simulink model "demoOtterUSVPathFollowingCourseControl"  (R2021a)
settings: Solver=ode4  StartTime=0.0  StopTime=300  FixedStep=0.05  RelTol=1e-3
libraries: mssSimulink x5, simulink x1
settings Model: Creator=thor  LastModifiedBy=Administrator

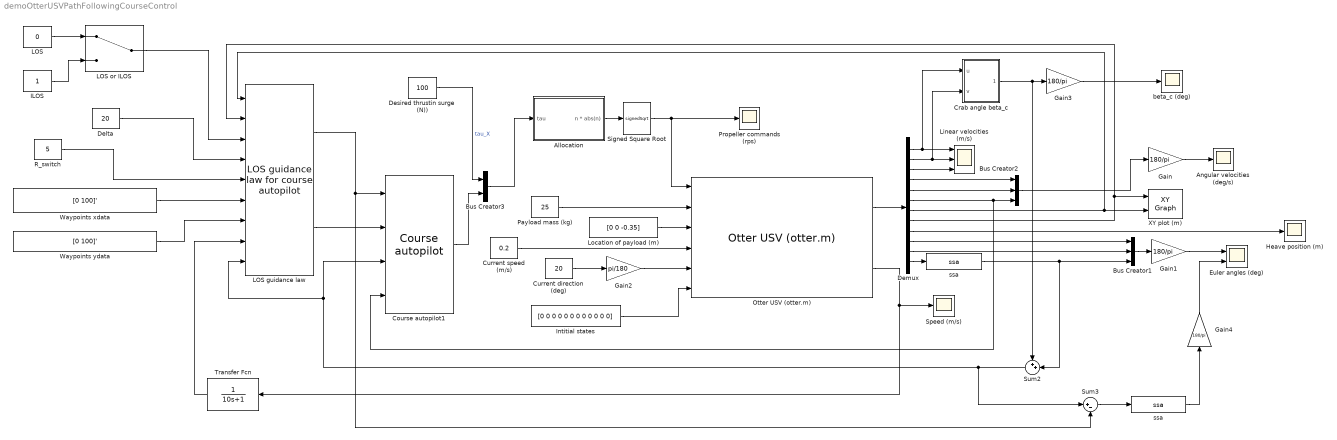
== system demoOtterUSVPathFollowingCourseControl ==
  Allocation : Subsystem
  Angular velocities (deg/s) : Scope
  Bus Creator1 : BusCreator  Inputs=3
  Bus Creator2 : BusCreator  Inputs=3
  Bus Creator3 : BusCreator  Inputs=2
  "Course autopilot1 " : mssSimulink/Control/Autopilots/Course autopilot  wn=1.2  zeta=1  T_nomoto=0.5  m=37.1
  Crab angle beta_c : Subsystem
  Current direction (deg) : Constant  Value=20
  Current speed (m/s) : Constant  Value=0.2
  Delta : Constant  Value=20
  Demux : Demux  Outputs=12
  Desired thrustin surge (N)) : Constant  Value=100
  Euler angles (deg) : Scope  NumInputPorts=2
  Gain{,1,3..4} (4 alike) : Gain  Gain=180/pi
  Gain2 : Gain  Gain=pi/180
  Heave position (m) : Scope
  ILOS : Constant
  Intitial states : Constant  Value=[0 0 0 0 0 0 0 0 0 0 0 0]
  LOS : Constant  Value=0
  LOS guidance law : mssSimulink/Guidance/LOS guidance law for course autopilot  SystemSampleTime=-1  VariantActivationTime=update diagram  Latency=0  AutoFrameSizeCalculation=off
  LOS or ILOS : ManualSwitch
  Linear velocities (m/s) : Scope  NumInputPorts=3
  Location of payload (m) : Constant  Value=[0 0 -0.35]
  "Otter USV (otter.m) " : mssSimulink/Marine craft models/Otter USV (otter.m)  SystemSampleTime=-1  VariantActivationTime=update diagram  Latency=0  AutoFrameSizeCalculation=off
  Payload mass (kg) : Constant  Value=25
  Propeller commands (rps) : Scope
  R_switch : Constant  Value=5
  Signed Square Root : Sqrt  Operator=signedSqrt  SaturateOnIntegerOverflow=on
  Speed (m/s) : Scope
  Sum2 : Sum  Inputs=++|  InputSameDT=on  SaturateOnIntegerOverflow=on  OutDataTypeStr=Inherit: Same as first input
  Sum3 : Sum  Inputs=|+-  InputSameDT=on  SaturateOnIntegerOverflow=on  OutDataTypeStr=Inherit: Same as first input
  Transfer Fcn : TransferFcn  Denominator=[10 1]
  Waypoints xdata : Constant  Value=[0 100]'
  Waypoints ydata : Constant  Value=[0 100]'
  XY plot (m) : simulink/Sinks/XY Graph  xmin=-200  xmax=500  ymin=-100  ymax=500  st=-1
  beta_c (deg) : Scope
  "ssa " : mssSimulink/Utilities/Math Operations/ssa  SystemSampleTime=-1  VariantActivationTime=update diagram  Latency=0  AutoFrameSizeCalculation=off
  "ssa   " : mssSimulink/Utilities/Math Operations/ssa  SystemSampleTime=-1  VariantActivationTime=update diagram  Latency=0  AutoFrameSizeCalculation=off
  wires:
  Demux/1 -> Linear velocities (m/s)/1, Crab angle beta_c/1(u)
  Demux/2 -> Linear velocities (m/s)/2, Crab angle beta_c/2(v)
  Demux/3 -> Linear velocities (m/s)/3
  Demux/10 -> Bus Creator1/1
  Demux/11 -> Bus Creator1/2
  Demux/4 -> Bus Creator2/1
  Demux/5 -> Bus Creator2/2
  Bus Creator2/1 -> Gain/1
  Demux/9 -> Heave position (m)/1
  Payload mass (kg)/1 -> "Otter USV (otter.m) "/2
  Location of payload (m)/1 -> "Otter USV (otter.m) "/3
  Current speed (m/s)/1 -> "Otter USV (otter.m) "/4
  Current direction (deg)/1 -> Gain2/1
  Intitial states/1 -> "Otter USV (otter.m) "/6
  "Otter USV (otter.m) "/1 -> Demux/1
  "Otter USV (otter.m) "/2 -> Speed (m/s)/1, Transfer Fcn/1
  Gain/1 -> Angular velocities (deg/s)/1
  Gain1/1 -> Euler angles (deg)/1
  Gain2/1 -> "Otter USV (otter.m) "/5
  "Course autopilot1 "/1 -> Bus Creator3/2
  Demux/12 -> "ssa   "/1
  Demux/6 -> "Course autopilot1 "/4, Bus Creator2/3
  Desired thrustin surge (N))/1 -> Bus Creator3/1  "tau_X"
  Bus Creator1/1 -> Gain1/1
  R_switch/1 -> LOS guidance law/5
  Delta/1 -> LOS guidance law/4
  Demux/7 -> LOS guidance law/1, XY plot (m)/2
  Demux/8 -> LOS guidance law/2, XY plot (m)/1
  Waypoints xdata/1 -> LOS guidance law/6
  Waypoints ydata/1 -> LOS guidance law/7
  Gain3/1 -> beta_c (deg)/1
  Transfer Fcn/1 -> LOS guidance law/8
  Sum3/1 -> "ssa "/1
  "ssa "/1 -> Gain4/1
  Gain4/1 -> Euler angles (deg)/2
  "ssa   "/1 -> Bus Creator1/3, Sum2/2
  LOS/1 -> LOS or ILOS/1
  ILOS/1 -> LOS or ILOS/2
  LOS or ILOS/1 -> LOS guidance law/3
  Sum2/1 -> Sum3/1, LOS guidance law/9, "Course autopilot1 "/3
  Allocation/1(n * abs(n)) -> Signed Square Root/1
  Bus Creator3/1 -> Allocation/1(tau)
  Signed Square Root/1 -> Propeller commands (rps)/1, "Otter USV (otter.m) "/1
  LOS guidance law/1 -> "Course autopilot1 "/1, Sum3/2
  LOS guidance law/2 -> "Course autopilot1 "/2
  Crab angle beta_c/1(beta_c) -> Gain3/1, Sum2/1

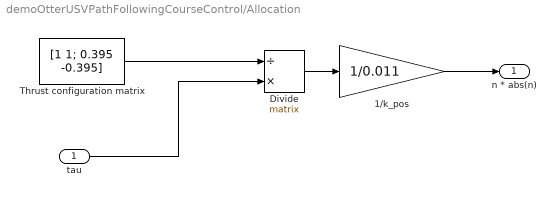
== system demoOtterUSVPathFollowingCourseControl/Allocation ==
  tau : Inport
  1/k_pos : Gain  Gain=1/0.011
  Divide : Product  Inputs=/*  Multiplication=Matrix(*)
  Thrust configuration matrix : Constant  Value=[1 1; 0.395 -0.395]
  n * abs(n) : Outport
  wires:
  1/k_pos/1 -> n * abs(n)/1
  tau/1 -> Divide/2
  Divide/1 -> 1/k_pos/1
  Thrust configuration matrix/1 -> Divide/1

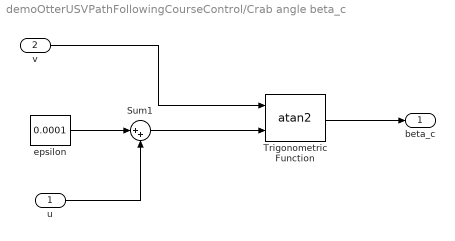
== system demoOtterUSVPathFollowingCourseControl/Crab angle beta_c ==
  u : Inport
  v : Inport  Port=2
  Sum1 : Sum  Inputs=|++  InputSameDT=on  SaturateOnIntegerOverflow=on  OutDataTypeStr=Inherit: Same as first input
  Trigonometric Function : Trigonometry  Operator=atan2
  epsilon : Constant  Value=0.0001
  beta_c : Outport
  wires:
  Trigonometric Function/1 -> beta_c/1
  v/1 -> Trigonometric Function/1
  Sum1/1 -> Trigonometric Function/2
  u/1 -> Sum1/2
  epsilon/1 -> Sum1/1
